simulink model "dynamicsValidationSim"  (R2018b)
settings: Solver=FixedStepDiscrete  StartTime=0.0  StopTime=179  FixedStep=0.1  RelTol=1e-3  EnableMultiTasking=on
libraries: BasicAircraftDynamicsBlock x1, NominalTrajectory x1
settings Model: Creator=JO20596  LastModifiedBy=BI28030
settings DataIOCC: LimitDataPoints=on  SaveFormat=Array  SignalLoggingSaveFormat=ModelDataLogs
settings OptimizationCC: ExpressionDepthLimit=2147483647  LifeSpan=inf
settings DebuggingCC: UnderspecifiedInitializationDetection=Classic  MergeDetectMultiDrivingBlocksExec=none  SolverPrmCheckMsg=warning  FcnCallInpInsideContextMsg=warning  StateNameClashWarn=warning  SFUnexpectedBacktrackingDiag=warning  SFNoUnconditionalDefaultTransitionDiag=warning  SFExecutionAtInitializationDiag=none
settings HardwareCC: ProdBitPerPointer=32  ProdBitPerSizeT=32  ProdBitPerPtrDiffT=32  ProdLargestAtomicFloat=None  ProdIntDivRoundTo=Undefined  ProdEndianess=Unspecified  ProdWordSize=32  ProdHWDeviceType=32-bit Generic
settings ModelReferenceCC: PropagateSignalLabelsOutOfModel=off
settings SFSimCC: SimUseLocalCustomCode=off
settings RTWCC: RTWUseLocalCustomCode=off
settings CodeAppCC: StateflowObjectComments=on
settings GRTTargetCC: TargetLangStandard=C89/C90 (ANSI)  GeneratePreprocessorConditionals=Disable all  CombineOutputUpdateFcns=off  GRTInterface=on
settings ConfigComp: CovMetricSettings=dw  CovHtmlReporting=on  CovSaveCumulativeToWorkspaceVar=on  CovSaveSingleToWorkspaceVar=on  CovExternalEMLEnable=off

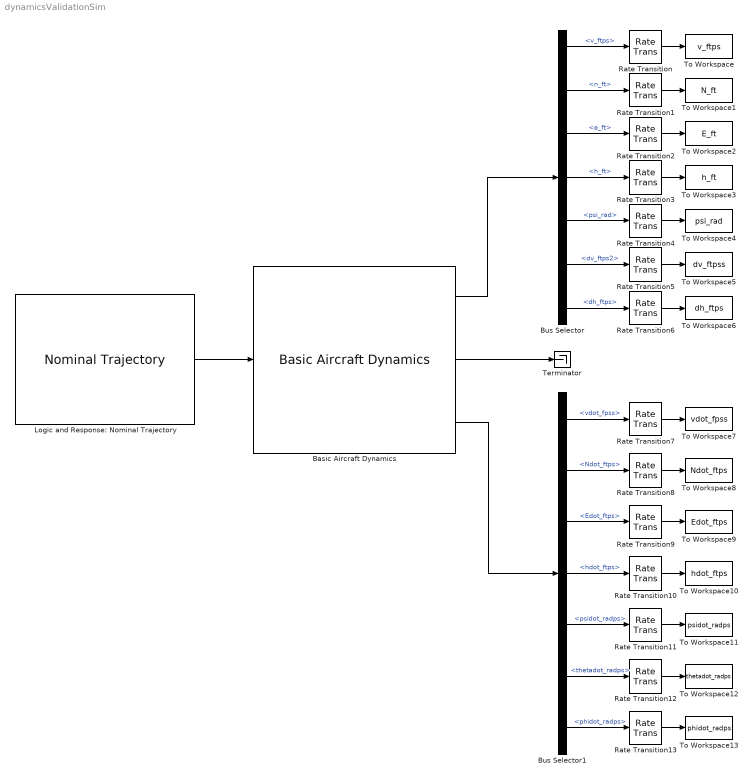
== system dynamicsValidationSim ==
  Basic Aircraft Dynamics : BasicAircraftDynamicsBlock/Basic Aircraft Dynamics  ts_dynamics=.1  v_ftps_0=ac1dyn_v_ftps  N_ft_0=ac1dyn_N_ft  E_ft_0=ac1dyn_E_ft  h_ft_0=ac1dyn_h_ft  psi_rad_0=ac1dyn_psi_rad  theta_rad_0=ac1dyn_theta_rad  phi_rad_0=ac1dyn_phi_rad  a_ftpss_0=ac1dyn_a_ftpss  v_ftps_max=ac1dyn_con.maxAirspeed_ftps  v_ftps_min=ac1dyn_con.minAirspeed_ftps  dv_ftpss_max=ac1dyn_con.maxAcceleration_ftpss  dv_ftpss_min=ac1dyn_con.minAcceleration_ftpss  dh_ftps_max=ac1dyn_con.maxVerticalRate_ftps  dh_ftps_min=ac1dyn_con.minVerticalRate_ftps  q_radps_max=ac1dyn_con.maxPitchRate_radps  phi_rad_max=ac1dyn_con.maxBankAngle_rad  dphi_radps_max=ac1dyn_con.maxRollRate_radps  r_radps_max=ac1dyn_con.maxYawRate_radps  pNUM=ac1dyn_con.dynamicsNumeratorRollRate  pDEN=ac1dyn_con.dynamicsDenominatorRollRate  hNUM=ac1dyn_con.dynamicsNumeratorVerticalRate  hDEN=ac1dyn_con.dynamicsDenominatorVerticalRate  rNUM=ac1dyn_con.dynamicsNumeratorYawRate  rDEN=ac1dyn_con.dynamicsDenominatorYawRate  lat0_rad=ac1dyn_lat0_rad  lon0_rad=ac1dyn_lon0_rad  alt_ft=ac1dyn_alt0_ft
  Bus Selector : BusSelector  OutputSignals=v_ftps,n_ft,e_ft,h_ft,psi_rad,dv_ftps2,dh_ftps
  Bus Selector1 : BusSelector  OutputSignals=vdot_fpss,Ndot_ftps,Edot_ftps,hdot_ftps,psidot_radps,thetadot_radps,phidot_radps
  Logic and Response: Nominal Trajectory : NominalTrajectory/Nominal Trajectory  eventFilename=event1.mat  ts=.1
  Rate Transition{,1..13} (14 alike) : RateTransition  OutPortSampleTime=1
  Terminator : Terminator
  To Workspace : ToWorkspace  VariableName=v_ftps  SampleTime=1
  To Workspace1 : ToWorkspace  VariableName=N_ft  SampleTime=1
  To Workspace10 : ToWorkspace  VariableName=hdot_ftps  SampleTime=-1
  To Workspace11 : ToWorkspace  VariableName=psidot_radps  SampleTime=-1
  To Workspace12 : ToWorkspace  VariableName=thetadot_radps  SampleTime=-1
  To Workspace13 : ToWorkspace  VariableName=phidot_radps  SampleTime=-1
  To Workspace2 : ToWorkspace  VariableName=E_ft  SampleTime=1
  To Workspace3 : ToWorkspace  VariableName=h_ft  SampleTime=1
  To Workspace4 : ToWorkspace  VariableName=psi_rad  SampleTime=1
  To Workspace5 : ToWorkspace  VariableName=dv_ftpss  SampleTime=1
  To Workspace6 : ToWorkspace  VariableName=dh_ftps  SampleTime=1
  To Workspace7 : ToWorkspace  VariableName=vdot_fpss  SampleTime=-1
  To Workspace8 : ToWorkspace  VariableName=Ndot_ftps  SampleTime=-1
  To Workspace9 : ToWorkspace  VariableName=Edot_ftps  SampleTime=-1
  wires:
  Basic Aircraft Dynamics/1 -> Bus Selector/1
  Bus Selector/1 -> Rate Transition/1  "<v_ftps>"
  Bus Selector/2 -> Rate Transition1/1  "<n_ft>"
  Bus Selector/3 -> Rate Transition2/1  "<e_ft>"
  Bus Selector/4 -> Rate Transition3/1  "<h_ft>"
  Bus Selector/5 -> Rate Transition4/1  "<psi_rad>"
  Rate Transition/1 -> To Workspace/1
  Rate Transition1/1 -> To Workspace1/1
  Rate Transition2/1 -> To Workspace2/1
  Rate Transition3/1 -> To Workspace3/1
  Rate Transition4/1 -> To Workspace4/1
  Rate Transition5/1 -> To Workspace5/1
  Bus Selector/6 -> Rate Transition5/1  "<dv_ftps2>"
  Rate Transition6/1 -> To Workspace6/1
  Bus Selector/7 -> Rate Transition6/1  "<dh_ftps>"
  Logic and Response: Nominal Trajectory/1 -> Basic Aircraft Dynamics/1
  Basic Aircraft Dynamics/2 -> Terminator/1
  Basic Aircraft Dynamics/3 -> Bus Selector1/1
  Bus Selector1/1 -> Rate Transition7/1  "<vdot_fpss>"
  Bus Selector1/2 -> Rate Transition8/1  "<Ndot_ftps>"
  Bus Selector1/3 -> Rate Transition9/1  "<Edot_ftps>"
  Bus Selector1/4 -> Rate Transition10/1  "<hdot_ftps>"
  Bus Selector1/5 -> Rate Transition11/1  "<psidot_radps>"
  Bus Selector1/6 -> Rate Transition12/1  "<thetadot_radps>"
  Bus Selector1/7 -> Rate Transition13/1  "<phidot_radps>"
  Rate Transition7/1 -> To Workspace7/1
  Rate Transition8/1 -> To Workspace8/1
  Rate Transition9/1 -> To Workspace9/1
  Rate Transition10/1 -> To Workspace10/1
  Rate Transition11/1 -> To Workspace11/1
  Rate Transition13/1 -> To Workspace13/1
  Rate Transition12/1 -> To Workspace12/1
